simulink model "queuetest_sixth"  (R2018a)
settings: Solver=VariableStepDiscrete  StartTime=0.0  StopTime=20.0  RelTol=1e-3
values from neighbouring files (symbols this model uses):
  LastHandle = Simulink.Parameter    [queuetest_sixth_multisim.m]
  LastQueue = Simulink.Parameter    [queuetest_sixth_multisim.m]
  TimeInSec = Simulink.Parameter    [queuetest_sixth_multisim.m]
undefined symbols (not defined in the file or in its folder): ControlModes, m, n
settings Model: Creator=Michael Girbino  LastModifiedBy=Michael Girbino
settings DebuggingCC: SFNoUnconditionalDefaultTransitionDiag=warning  SFOutputUsedAsStateInMooreChartDiag=warning

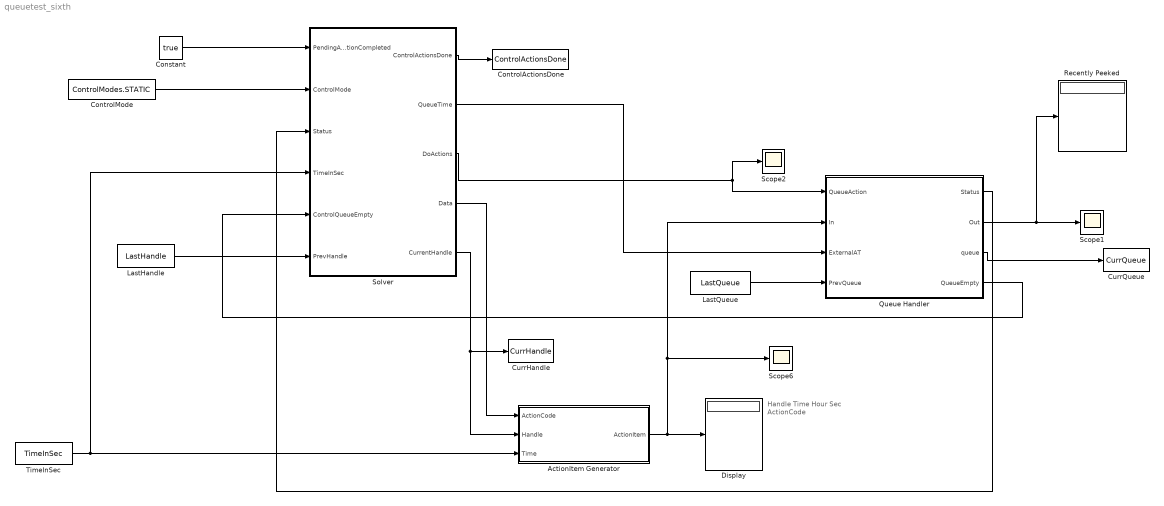
== system queuetest_sixth ==
  note: Handle
      | Time
      | Hour
      | Sec
      | ActionCode
  ActionItem Generator : Subsystem
  Constant : Constant  Value=true  OutDataTypeStr=boolean
  ControlActionsDone : ToWorkspace  VariableName=ControlActionsDone  SaveFormat=Timeseries  SampleTime=-1
  ControlMode : Constant  Value=ControlModes.STATIC  OutDataTypeStr=Enum: ControlModes
  CurrHandle : ToWorkspace  VariableName=CurrHandle  SaveFormat=Timeseries  SampleTime=-1
  CurrQueue : ToWorkspace  VariableName=CurrQueue  SaveFormat=Structure With Time  SampleTime=1
  Display : Display
  LastHandle : Constant  Value=LastHandle  OutDataTypeStr=double
  LastQueue : Constant  Value=LastQueue  VectorParams1D=off  OutDataTypeStr=double
  Queue Handler : Stateflow chart  TreatAsAtomicUnit=on
  Recently Peeked : Display
  Scope1 : Scope
  Scope2 : Scope
  Scope6 : Scope
  Solver : Stateflow chart  TreatAsAtomicUnit=on
  TimeInSec : Constant  Value=TimeInSec  OutDataTypeStr=double
  wires:
  Solver/3(DoActions) -> Queue Handler/1(QueueAction), Scope2/1
  Queue Handler/1(Status) -> Solver/3(Status)
  Queue Handler/2(Out) -> Scope1/1, Recently Peeked/1
  Queue Handler/3(queue) -> CurrQueue/1
  Solver/2(QueueTime) -> Queue Handler/3(ExternalAT)
  ControlMode/1 -> Solver/2(ControlMode)
  ActionItem Generator/1(ActionItem) -> Scope6/1, Queue Handler/2(In), Display/1
  Solver/4(Data) -> ActionItem Generator/1(ActionCode)
  Constant/1 -> Solver/1(PendingActionCompleted)
  Solver/1(ControlActionsDone) -> ControlActionsDone/1
  Queue Handler/4(QueueEmpty) -> Solver/5(ControlQueueEmpty)
  TimeInSec/1 -> Solver/4(TimeInSec), ActionItem Generator/3(Time)
  LastHandle/1 -> Solver/6(PrevHandle)
  Solver/5(CurrentHandle) -> CurrHandle/1, ActionItem Generator/2(Handle)
  LastQueue/1 -> Queue Handler/4(PrevQueue)

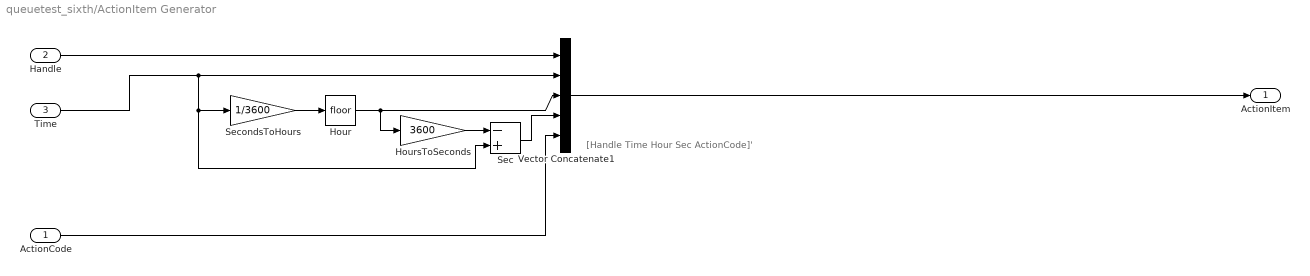
== system queuetest_sixth/ActionItem Generator ==
  note: [Handle Time Hour Sec ActionCode]'
  ActionCode : Inport
  Handle : Inport  Port=2
  Time : Inport  Port=3
  Hour : Rounding
  HoursToSeconds : Gain  Gain=3600
  Sec : Sum  Inputs=-+
  SecondsToHours : Gain  Gain=1/3600
  Vector Concatenate1 : Concatenate  NumInputs=5
  ActionItem : Outport
  wires:
  Time/1 -> Sec/2, SecondsToHours/1, Vector Concatenate1/2
  Hour/1 -> Vector Concatenate1/3, HoursToSeconds/1
  SecondsToHours/1 -> Hour/1
  Vector Concatenate1/1 -> ActionItem/1
  HoursToSeconds/1 -> Sec/1
  Handle/1 -> Vector Concatenate1/1
  Sec/1 -> Vector Concatenate1/4
  ActionCode/1 -> Vector Concatenate1/5

== stateflow chart queuetest_sixth/Solver ==
  state ControlFlow
    state SayPush
      en:
      Data = ii;
      DoActions.data = ...
      QueueActions.PUSH;
      send(DoActions);
      ii = ii+1;
      CurrentHandle = ...
      CurrentHandle + 1;
    note: Static
        | - dummy QueueTime
        | - DoNearestActions
    note: Event-driven
        | - QueueTime is current time
        | - DoNearestActions
    note: Time-driven
        | - QueueTime is current time
        | - DoActions
    note: Multirate
        | - QueueTime is current time
        | - DoMultiRate
    (default) -> SayPush : {CurrentHandle = PrevHandle;}
    (junction 103) -> SayPush [order 1] : [ii <= 10]
    SayPush -> (junction 25) [order 2] : Status[Status.data == Statuses.ERROR]
    SayPush -> (junction 103) [order 1] : Status[Status.data == Statuses.READY]
    (junction 103) -> (junction 25) [order 2]
    (junction 25) -> (junction 26) [order 1] : [ControlMode == ControlModes.STATIC]
    (junction 25) -> (junction 29) [order 2]
    (junction 26) -> (junction 54)
    (junction 54) -> (junction 55) [order 1] : [LocalControlQueueEmpty]
        | % execute nearest set of control actions, but leave time where it is
    (junction 54) -> (junction 56) [order 2] : {QueueTime = 0; %[0 0] xHour, xSec
        | DoActions.data = QueueActions.DO_NEAREST_ACTIONS;
        | send(DoActions);
        | % ignores time advancement
        | }
    (junction 55) -> (junction 57) : {ControlActionsDone = true;}
    (junction 57) -> (junction 56)
    (junction 56) -> (junction 27)
    (junction 27) -> (junction 28)
    (junction 28) -> (junction 32)
    (junction 29) -> (junction 30) [order 1] : [ControlMode == ControlModes.EVENTDRIVEN]
        | % execute nearest set of control actions and advance time to that time
    (junction 30) -> (junction 65) : {QueueTime = TimeInSec; %xHour, xSec
        | DoActions.data = QueueActions.DO_NEAREST_ACTIONS;
        | send(DoActions);}
    (junction 29) -> (junction 33) [order 2]
    (junction 65) -> (junction 66) [order 1] : [~PendingActionCompleted]
    (junction 65) -> (junction 67) [order 2]
    (junction 66) -> (junction 68) : {ControlActionsDone = true;
        | % advances time to the next event
        | }
    (junction 68) -> (junction 67)
    (junction 67) -> (junction 31)
    (junction 31) -> (junction 32)
    (junction 32) -> (junction 36)
    (junction 33) -> (junction 34) [order 1] : [ControlMode == ControlModes.TIMEDRIVEN]
        |  % Do all actions having and action time <= specified time
    (junction 33) -> (junction 37) [order 2]
    (junction 34) -> (junction 78) : {QueueTime = TimeInSec; %xHour, xSec
        | DoActions.data = QueueActions.DO_ACTIONS;
        | send(DoActions);}
    (junction 78) -> (junction 80) [order 1] : [~PendingActionCompleted]
    (junction 78) -> (junction 79) [order 2]
    (junction 80) -> (junction 82) : {ControlActionsDone = true;
        | }
    (junction 82) -> (junction 79)
    (junction 79) -> (junction 35)
    (junction 35) -> (junction 36)
    (junction 36) -> (junction 40)
    (junction 37) -> (junction 38) [order 1] : [ControlMode == ControlModes.MULTIRATE]
        |  % Execute the nearest set of control actions, but leave time where it is
    (junction 37) -> (junction 41) [order 2]
    (junction 38) -> (junction 91) : {QueueTime =TimeInSec; %xHour, xSec
        | DoActions.data = QueueActions.DO_MULTIRATE;
        | send(DoActions);}
    (junction 91) -> (junction 88) [order 1] : [~PendingActionCompleted]
    (junction 91) -> (junction 87) [order 2]
    (junction 88) -> (junction 92) : {ControlActionsDone = true;
        | }
    (junction 92) -> (junction 87)
    (junction 87) -> (junction 39)
    (junction 39) -> (junction 40)
    (junction 40) -> (junction 42)
    (junction 42) -> (junction 41)
    (junction 41) -> (junction 43)
  state QueueEmptyCase
    en: LocalControlQueueEmpty = true;
  (default) -> ControlFlow
  QueueEmptyCase -> ControlFlow
  ControlFlow -> QueueEmptyCase : ControlQueueEmpty
  data: ControlActionsDone output boolean; QueueTime output double; DoActions output Enum: QueueActions; PendingActionCompleted input boolean; ControlMode input Enum: ControlModes; Data output double size=1; ii local double =0; Status input Enum: Statuses; TimeInSec input double; LocalControlQueueEmpty local boolean =false; ControlQueueEmpty input boolean; PrevHandle input double; CurrentHandle output double

== stateflow chart queuetest_sixth/Queue Handler ==
  settings: enableNonTerminalStates=1
  state Executive [parallel]
    settings: executionOrder=1
    state Asleep
      ex: Status.data = Statuses.READY; % reset status
      INTERNAL_DONE = false;
      EXECUTIVE_DONE = false;
    state DoNearestActions
      state WaitOnPeek
        en: send(QUEUE_PEEK, Internal);
      state WaitOnPop
        en: send(QUEUE_POP, Internal);
      state ErrorNoItems
        en: Status.data = ...
        Statuses.ERROR;
        send(Status);
      (default) -> (junction 302) : % do only those actions with the same delay time as the first action time return time
          | {q_len_initial = GetQueueSize;
          | PendingActionsCompleted = false; % local for now
          | }
      (junction 302) -> (junction 315) [order 1] : [q_len_initial > 0]
      (junction 302) -> Executive.DoNearestActions.ErrorNoItems [order 2]
      (junction 315) -> WaitOnPeek : {INTERNAL_DONE = false;
          | ActionTime = ExternalAT; % peek with given AT
          | }
      (junction 301) -> (junction 331) [order 1] : [jj <= q_len_initial]
      (junction 331) -> Executive.DoNearestActions.WaitOnPop : {INTERNAL_DONE = false;}
      WaitOnPeek -> (junction 301) : [INTERNAL_DONE]
          | {ActionTime = Out(QF.Time);
          | QHour = Out(QF.Hour);
          | QSec = Out(QF.Sec);
          | jj = 1;}
      Executive.DoNearestActions.WaitOnPop -> (junction 299) : [INTERNAL_DONE]
          | %send(DoPendingAction);
      (junction 299) -> (junction 301) : {jj = jj + 1;}
      (junction 301) -> (junction 305) [order 2]
      Executive.DoNearestActions.ErrorNoItems -> (junction 300)
      (junction 305) -> (junction 300)
      (junction 300) -> (junction 298) : {EXECUTIVE_DONE = true;}
    state DoAllActions
      state WaitOnPop
        en: send(QUEUE_POP, Internal);
      state ErrorNoItems
        en: Status.data = ...
        Statuses.ERROR;
        send(Status);
      (default) -> (junction 322) : {q_len_initial = GetQueueSize;}
      (junction 322) -> (junction 321) [order 1] : [q_len_initial ~= 0]
      (junction 322) -> Executive.DoAllActions.ErrorNoItems [order 2]
      (junction 321) -> (junction 326) : {ActionTime = ExternalAT;
          | jj = 1;}
      (junction 326) -> (junction 316) [order 1] : [jj <= q_len_initial]
      (junction 316) -> Executive.DoAllActions.WaitOnPop : {INTERNAL_DONE = false;}
      (junction 314) -> (junction 326) : {jj = jj + 1;}
      (junction 326) -> (junction 312) [order 2]
      Executive.DoAllActions.WaitOnPop -> (junction 314) : [INTERNAL_DONE]
          | %send(DoPendingAction);
      Executive.DoAllActions.ErrorNoItems -> (junction 324)
      (junction 312) -> (junction 324)
      (junction 324) -> (junction 310) : {EXECUTIVE_DONE = true;}
    state Pushing
      en: send(QUEUE_PUSH, Internal);
    state Peeking
      en: send(QUEUE_PEEK, Internal);
    state Popping
      en: send(QUEUE_POP, Internal);
    state ReadyAgain
      Status.data = Statuses.READY;
      send(Status);
    Executive.Asleep -> Executive.Peeking [order 5] : QueueAction[QueueAction.data == ...
        | QueueActions.PEEK]
    Executive.Asleep -> Executive.Popping [order 4] : QueueAction[QueueAction.data == ...
        | QueueActions.POP]
    (default) -> Executive.Asleep
    Executive.Asleep -> Executive.Pushing [order 3] : QueueAction[QueueAction.data == ...
        | QueueActions.PUSH]
    Executive.Asleep -> DoAllActions [order 2] : QueueAction[QueueAction.data == ...
        | QueueActions.DO_ALL_ACTIONS]
    ReadyAgain -> Executive.Asleep
    Executive.Asleep -> DoNearestActions [order 1] : QueueAction[QueueAction.data == DO_NEAREST_ACTIONS]
    Executive.Pushing -> ReadyAgain : [INTERNAL_DONE]
    Executive.Popping -> ReadyAgain : [INTERNAL_DONE]
    Executive.Peeking -> ReadyAgain : [INTERNAL_DONE]
    DoAllActions -> ReadyAgain : [EXECUTIVE_DONE]
    DoNearestActions -> ReadyAgain : [EXECUTIVE_DONE]
  state Internal [parallel]
    settings: executionOrder=2
    state Asleep
    state Popping
      (default) -> (junction 163) : % delete from beginning, t<= ActionTime:
          | {q_len = GetQueueSize;
          | ii = 1;
          | }
      (junction 163) -> (junction 169) [order 1] : [ii <= q_len]
      (junction 169) -> (junction 157)
      (junction 157) -> (junction 158) [order 1] : [GetElemTime(ii) <= ActionTime]
      (junction 157) -> (junction 164) [order 2]
      (junction 158) -> (junction 159) : {Out = GetElem(ii);
          | ReduceQueue(ii);}
          | % break
      (junction 164) -> (junction 163) : {ii = ii + 1;}
      (junction 163) -> (junction 165) [order 2]
      (junction 159) -> (junction 165)
      (junction 165) -> (junction 640)
      (junction 640) -> (junction 641) [order 1] : [QueueEmpty.data == true]
      (junction 640) -> (junction 642) [order 2]
      (junction 641) -> (junction 643) : {send(QueueEmpty);}
      (junction 643) -> (junction 642)
      (junction 642) -> (junction 644) : {INTERNAL_DONE = true;}
    state Pushing
      (default) -> (junction 136) : % insert into queue right before item of greater or equal execution time
          | {q_cand = In'; % transposition to 1 x 5
          | q_len = GetQueueSize; %size(queue, 3);
          | ii = 1;
          | }
      (junction 136) -> (junction 134) [order 1] : [ii <= q_len]
      (junction 134) -> (junction 145)
      (junction 145) -> (junction 146) [order 1] : [q_cand(1,QF.Time) <= GetElemTime(ii)]
      (junction 145) -> (junction 137) [order 2]
      (junction 146) -> (junction 148) : {
          | ExpandQueue(ii);}
          | % break
      (junction 137) -> (junction 136) : {ii = ii + 1;}
      (junction 136) -> (junction 138) [order 2] : {ExpandQueue(q_len+1);}
      (junction 148) -> (junction 138)
      (junction 138) -> (junction 151) : %{send(DONE_PUSHING, Executive.Pushing);}
          | {INTERNAL_DONE = true;}
    state Peeking
      (default) -> (junction 181) : % pop without deletion
          | {q_len = GetQueueSize;
          | ii = 1;
          | }
      (junction 181) -> (junction 187) [order 1] : [ii <= q_len]
      (junction 187) -> (junction 175)
      (junction 175) -> (junction 176) [order 1] : [GetElemTime(ii) <= ActionTime]
      (junction 175) -> (junction 182) [order 2]
      (junction 176) -> (junction 177) : {Out = GetElem(ii);}
          | % break
      (junction 182) -> (junction 181) : {ii = ii + 1;}
      (junction 181) -> (junction 183) [order 2]
      (junction 177) -> (junction 183)
      (junction 183) -> (junction 180) : {INTERNAL_DONE = true;}
    (default) -> Internal.Asleep
    Internal.Asleep -> Internal.Pushing [order 1] : QUEUE_PUSH
    Internal.Pushing -> Internal.Asleep : [INTERNAL_DONE]
    Internal.Asleep -> Internal.Popping [order 2] : QUEUE_POP
    Internal.Popping -> Internal.Asleep : [INTERNAL_DONE]
    Internal.Asleep -> Internal.Peeking [order 3] : QUEUE_PEEK
    Internal.Peeking -> Internal.Asleep : [INTERNAL_DONE]
  state QF % Queue Fields [group]
  state qs = GetQueueSize [function]
    (default) -> (junction 649) : {[qs, QueueEmpty.data] = mlGetQueueSize;}
  data: Handle local double =1; Time local double =2; Hour local double =3; Sec local double =4; ActionCode local double =5; qs function_output; q_size function_output; qe_data function_output; depth function_input; et function_output; elem function_output; depth function_input; depth function_input; depth function_input; QueueAction input Enum: QueueActions; Status output Enum: Statuses; Out output double size=[1 5] =zeros(1,5); queue output double size=[1 5 50]; q_len local double =0; PendingActionsCompleted local boolean =false; QHour local double; QSec local double; q_cand local double size=[1 5]; In input double size=5; qwriteflag local boolean =false; ii local uint8; jj local uint8; q_len_initial local double; EXECUTIVE_DONE local boolean =false; INTERNAL_DONE local boolean =false;; ExternalAT input double =100; ActionTime local double; QueueEmpty output boolean =false; PrevQueue input double size=[1 5 50]
  events: QUEUE_POP local FUNCTION_CALL_EVENT; QUEUE_PUSH local FUNCTION_CALL_EVENT; QUEUE_PEEK local FUNCTION_CALL_EVENT
  function [q_size, qe_data] = mlGetQueueSize:
    | function [q_size, qe_data] = mlGetQueueSize
    | %     coder.extrinsic('exist');
    | %     eq = zeros(1,1,'double');
    | %     eq = exist('queue');
    | %     if eq == 1 && ~isempty(queue)
    | %         qs = size(queue, 3);
    | %     else % eq ~= 1 || size == 0
    | %         qs = 0;
    | %     end
    |     if ~qwriteflag % can't read intial value of empty queue, so depend on flag
    |         % queue = zeros(1,5);
    |         queue = PrevQueue;
    |         q_size = 0;
    |         qe_data = true;
    |         %QueueEmpty.data = true;
    |         qwriteflag = true;
    |     elseif isequal(queue,zeros(1,5)) % case of empty queue (still 1 element)
    |         q_size = 0;
    |         qe_data = true;
    |         %QueueEmpty.data = true;
    |     else
    |         q_size = size(queue,3);
    |         qe_data = false;
    |         %QueueEmpty.data = false;
    |     end
    | end
  function et = GetElemTime(depth):
    | function et = GetElemTime(depth)
    |     et = zeros(1,1);
    |     if ~isempty(queue)
    |         et = queue(1,QF.Time,ii);
    |     else
    |     end
    | end
  function elem = GetElem(depth):
    | function elem = GetElem(depth)
    |     elem = zeros(1,5);
    |     elem(1,:) = queue(:,:,depth);
    | end
  function ExpandQueue(depth):
    | function ExpandQueue(depth)
    |     rhs = queue(:,:,depth:q_len); % the RHS of the queue
    |     bigger = zeros(1,5,q_len+1);
    |     bigger(:,:,1:(depth-1)) = queue(:,:,1:(depth-1)); % copy LHS
    |     bigger(:,:,depth) = q_cand; % inserting element at end of LHS
    |     %queue(:,:,depth) = q_cand; 
    |     bigger(:,:, (depth+1):(q_len+1)) = rhs; % tack on RHS again
    |     queue = bigger;
    | end
  function ReduceQueue(depth):
    | function ReduceQueue(depth)
    |     rhs = queue(:,:,(depth+1):q_len); % excluding element at depth
    |     smaller = zeros(1,5,q_len-1);
    |     smaller(:,:,1:(depth-1)) = queue(:,:,1:(depth-1)); % lhs, excl. depth
    |     smaller(:,:,depth:(q_len-1)) = rhs; % tack on rhs
    |     queue = smaller;
    | end
